simulink model "DigitalTwin"  (R2023b)
settings: Solver=ode23t  StartTime=0.0  StopTime=600  RelTol=1e-3  AbsTol=1e-3
model workspace: external: MATLAB File C:\Users\claud\OneDrive - TUM\COME -TUM\Software lab\Three_wheeled_base\simscape_1\Three_wheeled_base_DataFile1.m (data not in the file)
values from neighbouring files (symbols this model uses):
  brick_pick_global_xy = [brick_pick_global_xy, new_column]    [Three_wheeled_base_LOAD_DATA.m]
  brick_place_global_xy = [brick_place_global_xy, new_column]    [Three_wheeled_base_LOAD_DATA.m]
  platform_destination_mat = [ 1.0 0; 5 0; 0 0; 0 5 ... (first row only)    [Three_wheeled_base_LOAD_DATA.m]
undefined symbols (not defined in the file or in its folder): robotData, smiData, X, Y, Z
libraries: sm_lib x237, nesl_utility x78, fl_lib x12, batteryecm_lib x5, ee_lib x3, robotcorelib x1, robotalgslib x1
(part 7 of 7)

== system DigitalTwin/Arm/Kinova Gen3 Arm/right_inner_knuckle ==
  Inertia : sm_lib/Body Elements/Inertia  InertiaType=Custom  Mass=0.0110930853895903  MassUnits=kg  CenterOfMass=[0, 0, 0]  CenterOfMassUnits=m  MomentsOfInertia=[4.27134775939882e-06, 3.96548790524392e-06, 3.20325997634666e-06]  MomentsOfInertiaUnits=kg*m^2  ProductsOfInertia=[-8.45108024914164e-15, 1.77774229944246e-06, -8.53568456728898e-15]  ProductsOfInertiaUnits=kg*m^2  GraphicType=None  MarkerShape=Inertia  MarkerSize=20  GraphicVisPropType=SimpleVisualProperties  GraphicDiffuseColor=[0.5 0.5 0.5]  GraphicSpecularColor=[0.5 0.5 0.5 1.0]  GraphicAmbientColor=[0.15 0.15 0.15 1.0]  GraphicEmissiveColor=[0.0 0.0 0.0 1.0]  GraphicShininess=75  GraphicOpacity=1.0
  InertiaOriginTransform : sm_lib/Frames and Transforms/Rigid Transform  TranslationMethod=Cartesian  TranslationStandardOffset=0  TranslationStandardOffsetUnits=m  TranslationStandardAxis=+Z  TranslationCartesianOffset=[0.0168606186773776, 3.93808471820465e-10, 0.0226699950793434]  TranslationCartesianOffsetUnits=m  TranslationROffset=0  TranslationROffsetUnits=m  TranslationZOffset=0  TranslationZOffsetUnits=m  TranslationThetaOffset=0  TranslationThetaOffsetUnits=deg  RotationMethod=RotationSequence  RotationAngleUnits=deg  RotationStandardAxis=+Z  RotationAngle=0.0  RotationArbitraryAxis=[0 0 1]  FollAlignAxisA=+X  BaseAlignAxisA=+Y  FollAlignAxisB=+Y  BaseAlignAxisB=+Z  RotationSequenceAxes=BaseAxes  RotationSequence=XYZ  RotationSequenceAngles=[0, 0, 0]  RotationSequenceAnglesUnits=rad  RotationMatrix=[1 0 0; 0 1 0; 0 0 1]  Quaternion=[1 0 0 0]
  ReferenceFrame : sm_lib/Frames and Transforms/Reference Frame
  Visual : sm_lib/Body Elements/File Solid  ExtGeomFileName=Gripper85\inner_knuckle_fine.STL  UnitType=Custom  ExtGeomFileUnits=m  StepReaderType=HEX  ExportConvexHullGeometry=off  InertiaType=Custom  Mass=0  MassUnits=kg  CenterOfMass=[0, 0, 0]  CenterOfMassUnits=m  MomentsOfInertia=[0, 0, 0]  MomentsOfInertiaUnits=kg*m^2  ProductsOfInertia=[0, 0, 0]  ProductsOfInertiaUnits=kg*m^2  BasedOnType=DensityFromFile  Density=1000  DensityUnits=kg/m^3  DoExposeReferenceFrame=on  SerializedFrames=<Frames/>  GraphicType=FromGeometry  MarkerShape=Sphere  MarkerSize=10  GraphicVisPropType=SimpleVisualProperties  GraphicDiffuseColor=[0.1, 0.1, 0.1]  GraphicSpecularColor=[0.5 0.5 0.5 1.0]  GraphicAmbientColor=[0.15 0.15 0.15 1.0]  GraphicEmissiveColor=[0.0 0.0 0.0 1.0]  GraphicShininess=75  GraphicOpacity=1
  VisualOriginTransform : sm_lib/Frames and Transforms/Rigid Transform  TranslationMethod=Cartesian  TranslationStandardOffset=0  TranslationStandardOffsetUnits=m  TranslationStandardAxis=+Z  TranslationCartesianOffset=[0, 0, 0]  TranslationCartesianOffsetUnits=m  TranslationROffset=0  TranslationROffsetUnits=m  TranslationZOffset=0  TranslationZOffsetUnits=m  TranslationThetaOffset=0  TranslationThetaOffsetUnits=deg  RotationMethod=RotationSequence  RotationAngleUnits=deg  RotationStandardAxis=+Z  RotationAngle=0.0  RotationArbitraryAxis=[0 0 1]  FollAlignAxisA=+X  BaseAlignAxisA=+Y  FollAlignAxisB=+Y  BaseAlignAxisB=+Z  RotationSequenceAxes=BaseAxes  RotationSequence=XYZ  RotationSequenceAngles=[0, 0, 0]  RotationSequenceAnglesUnits=rad  RotationMatrix=[1 0 0; 0 1 0; 0 0 1]  Quaternion=[1 0 0 0]
  right_inner_finger_joint_AxisTransform : sm_lib/Frames and Transforms/Rigid Transform  TranslationMethod=Cartesian  TranslationStandardOffset=0  TranslationStandardOffsetUnits=m  TranslationStandardAxis=+Z  TranslationCartesianOffset=[0, 0, 0]  TranslationCartesianOffsetUnits=m  TranslationROffset=0  TranslationROffsetUnits=m  TranslationZOffset=0  TranslationZOffsetUnits=m  TranslationThetaOffset=0  TranslationThetaOffsetUnits=deg  RotationMethod=ArbitraryAxis  RotationAngleUnits=rad  RotationStandardAxis=+Z  RotationAngle=1.570796326794897  RotationArbitraryAxis=[-1, 0, 0]  FollAlignAxisA=+X  BaseAlignAxisA=+Y  FollAlignAxisB=+Y  BaseAlignAxisB=+Z  RotationSequenceAxes=FollowerAxes  RotationSequence=XYX  RotationSequenceAngles=[0 0 0]  RotationSequenceAnglesUnits=deg  RotationMatrix=[1 0 0; 0 1 0; 0 0 1]  Quaternion=[1 0 0 0]
  right_inner_finger_joint_OriginTransform : sm_lib/Frames and Transforms/Rigid Transform  TranslationMethod=Cartesian  TranslationStandardOffset=0  TranslationStandardOffsetUnits=m  TranslationStandardAxis=+Z  TranslationCartesianOffset=[0.0341060475457406, 0, 0.0458573878541688]  TranslationCartesianOffsetUnits=m  TranslationROffset=0  TranslationROffsetUnits=m  TranslationZOffset=0  TranslationZOffsetUnits=m  TranslationThetaOffset=0  TranslationThetaOffsetUnits=deg  RotationMethod=RotationSequence  RotationAngleUnits=deg  RotationStandardAxis=+Z  RotationAngle=0.0  RotationArbitraryAxis=[0 0 1]  FollAlignAxisA=+X  BaseAlignAxisA=+Y  FollAlignAxisB=+Y  BaseAlignAxisB=+Z  RotationSequenceAxes=BaseAxes  RotationSequence=XYZ  RotationSequenceAngles=[0, 0, 0]  RotationSequenceAnglesUnits=rad  RotationMatrix=[1 0 0; 0 1 0; 0 0 1]  Quaternion=[1 0 0 0]
  right_inner_knuckle_joint_AxisInvTransform : sm_lib/Frames and Transforms/Rigid Transform  TranslationMethod=Cartesian  TranslationStandardOffset=0  TranslationStandardOffsetUnits=m  TranslationStandardAxis=+Z  TranslationCartesianOffset=[0, 0, 0]  TranslationCartesianOffsetUnits=m  TranslationROffset=0  TranslationROffsetUnits=m  TranslationZOffset=0  TranslationZOffsetUnits=m  TranslationThetaOffset=0  TranslationThetaOffsetUnits=deg  RotationMethod=ArbitraryAxis  RotationAngleUnits=rad  RotationStandardAxis=+Z  RotationAngle=1.570796326794897  RotationArbitraryAxis=[-1, 0, 0]  FollAlignAxisA=+X  BaseAlignAxisA=+Y  FollAlignAxisB=+Y  BaseAlignAxisB=+Z  RotationSequenceAxes=FollowerAxes  RotationSequence=XYX  RotationSequenceAngles=[0 0 0]  RotationSequenceAnglesUnits=deg  RotationMatrix=[1 0 0; 0 1 0; 0 0 1]  Quaternion=[1 0 0 0]
  F : PMIOPort  Side=Left
  F1 : PMIOPort  Port=2  Side=Right
  connections:
  Inertia/RConn1 -- InertiaOriginTransform/RConn1
  ReferenceFrame/RConn1 -- InertiaOriginTransform/LConn1 -- right_inner_finger_joint_OriginTransform/LConn1 -- right_inner_knuckle_joint_AxisInvTransform/LConn1 -- VisualOriginTransform/LConn1
  Visual/RConn1 -- VisualOriginTransform/RConn1
  right_inner_finger_joint_AxisTransform/RConn1 -- F1/RConn1
  right_inner_finger_joint_AxisTransform/LConn1 -- right_inner_finger_joint_OriginTransform/RConn1
  right_inner_knuckle_joint_AxisInvTransform/RConn1 -- F/RConn1

== system DigitalTwin/Arm/Kinova Gen3 Arm/right_outer_finger ==
  Inertia : sm_lib/Body Elements/Inertia  InertiaType=Custom  Mass=0.0273093985570947  MassUnits=kg  CenterOfMass=[0, 0, 0]  CenterOfMassUnits=m  MomentsOfInertia=[8.52366028592721e-06, 6.91333280651081e-06, 2.24270431912283e-06]  MomentsOfInertiaUnits=kg*m^2  ProductsOfInertia=[7.37726682706417e-19, 3.18003675694284e-07, 3.41683380899422e-19]  ProductsOfInertiaUnits=kg*m^2  GraphicType=None  MarkerShape=Inertia  MarkerSize=20  GraphicVisPropType=SimpleVisualProperties  GraphicDiffuseColor=[0.5 0.5 0.5]  GraphicSpecularColor=[0.5 0.5 0.5 1.0]  GraphicAmbientColor=[0.15 0.15 0.15 1.0]  GraphicEmissiveColor=[0.0 0.0 0.0 1.0]  GraphicShininess=75  GraphicOpacity=1.0
  InertiaOriginTransform : sm_lib/Frames and Transforms/Rigid Transform  TranslationMethod=Cartesian  TranslationStandardOffset=0  TranslationStandardOffsetUnits=m  TranslationStandardAxis=+Z  TranslationCartesianOffset=[0.00108844269639009, -2.611488350845e-15, 0.0215530225245502]  TranslationCartesianOffsetUnits=m  TranslationROffset=0  TranslationROffsetUnits=m  TranslationZOffset=0  TranslationZOffsetUnits=m  TranslationThetaOffset=0  TranslationThetaOffsetUnits=deg  RotationMethod=RotationSequence  RotationAngleUnits=deg  RotationStandardAxis=+Z  RotationAngle=0.0  RotationArbitraryAxis=[0 0 1]  FollAlignAxisA=+X  BaseAlignAxisA=+Y  FollAlignAxisB=+Y  BaseAlignAxisB=+Z  RotationSequenceAxes=BaseAxes  RotationSequence=XYZ  RotationSequenceAngles=[0, 0, 0]  RotationSequenceAnglesUnits=rad  RotationMatrix=[1 0 0; 0 1 0; 0 0 1]  Quaternion=[1 0 0 0]
  ReferenceFrame : sm_lib/Frames and Transforms/Reference Frame
  Visual : sm_lib/Body Elements/File Solid  ExtGeomFileName=Gripper85\outer_finger_fine.STL  UnitType=Custom  ExtGeomFileUnits=m  StepReaderType=HEX  ExportConvexHullGeometry=off  InertiaType=Custom  Mass=0  MassUnits=kg  CenterOfMass=[0, 0, 0]  CenterOfMassUnits=m  MomentsOfInertia=[0, 0, 0]  MomentsOfInertiaUnits=kg*m^2  ProductsOfInertia=[0, 0, 0]  ProductsOfInertiaUnits=kg*m^2  BasedOnType=DensityFromFile  Density=1000  DensityUnits=kg/m^3  DoExposeReferenceFrame=on  SerializedFrames=<Frames/>  GraphicType=FromGeometry  MarkerShape=Sphere  MarkerSize=10  GraphicVisPropType=SimpleVisualProperties  GraphicDiffuseColor=[0.1, 0.1, 0.1]  GraphicSpecularColor=[0.5 0.5 0.5 1.0]  GraphicAmbientColor=[0.15 0.15 0.15 1.0]  GraphicEmissiveColor=[0.0 0.0 0.0 1.0]  GraphicShininess=75  GraphicOpacity=1
  VisualOriginTransform : sm_lib/Frames and Transforms/Rigid Transform  TranslationMethod=Cartesian  TranslationStandardOffset=0  TranslationStandardOffsetUnits=m  TranslationStandardAxis=+Z  TranslationCartesianOffset=[0, 0, 0]  TranslationCartesianOffsetUnits=m  TranslationROffset=0  TranslationROffsetUnits=m  TranslationZOffset=0  TranslationZOffsetUnits=m  TranslationThetaOffset=0  TranslationThetaOffsetUnits=deg  RotationMethod=RotationSequence  RotationAngleUnits=deg  RotationStandardAxis=+Z  RotationAngle=0.0  RotationArbitraryAxis=[0 0 1]  FollAlignAxisA=+X  BaseAlignAxisA=+Y  FollAlignAxisB=+Y  BaseAlignAxisB=+Z  RotationSequenceAxes=BaseAxes  RotationSequence=XYZ  RotationSequenceAngles=[0, 0, 0]  RotationSequenceAnglesUnits=rad  RotationMatrix=[1 0 0; 0 1 0; 0 0 1]  Quaternion=[1 0 0 0]
  F : PMIOPort  Side=Left
  connections:
  Inertia/RConn1 -- InertiaOriginTransform/RConn1
  ReferenceFrame/RConn1 -- InertiaOriginTransform/LConn1 -- VisualOriginTransform/LConn1 -- F/RConn1
  Visual/RConn1 -- VisualOriginTransform/RConn1

== system DigitalTwin/Arm/Kinova Gen3 Arm/right_outer_knuckle ==
  Inertia : sm_lib/Body Elements/Inertia  InertiaType=Custom  Mass=0.00684838849401352  MassUnits=kg  CenterOfMass=[0, 0, 0]  CenterOfMassUnits=m  MomentsOfInertia=[2.70004361573169e-07, 1.38892332558312e-06, 1.26286103637978e-06]  MomentsOfInertiaUnits=kg*m^2  ProductsOfInertia=[2.82357800318817e-15, 1.56396493788199e-07, 1.59579467624491e-15]  ProductsOfInertiaUnits=kg*m^2  GraphicType=None  MarkerShape=Inertia  MarkerSize=20  GraphicVisPropType=SimpleVisualProperties  GraphicDiffuseColor=[0.5 0.5 0.5]  GraphicSpecularColor=[0.5 0.5 0.5 1.0]  GraphicAmbientColor=[0.15 0.15 0.15 1.0]  GraphicEmissiveColor=[0.0 0.0 0.0 1.0]  GraphicShininess=75  GraphicOpacity=1.0
  InertiaOriginTransform : sm_lib/Frames and Transforms/Rigid Transform  TranslationMethod=Cartesian  TranslationStandardOffset=0  TranslationStandardOffsetUnits=m  TranslationStandardAxis=+Z  TranslationCartesianOffset=[0.0178097074051638, 3.60493211424024e-11, 0.00233123458346721]  TranslationCartesianOffsetUnits=m  TranslationROffset=0  TranslationROffsetUnits=m  TranslationZOffset=0  TranslationZOffsetUnits=m  TranslationThetaOffset=0  TranslationThetaOffsetUnits=deg  RotationMethod=RotationSequence  RotationAngleUnits=deg  RotationStandardAxis=+Z  RotationAngle=0.0  RotationArbitraryAxis=[0 0 1]  FollAlignAxisA=+X  BaseAlignAxisA=+Y  FollAlignAxisB=+Y  BaseAlignAxisB=+Z  RotationSequenceAxes=BaseAxes  RotationSequence=XYZ  RotationSequenceAngles=[0, 0, 0]  RotationSequenceAnglesUnits=rad  RotationMatrix=[1 0 0; 0 1 0; 0 0 1]  Quaternion=[1 0 0 0]
  ReferenceFrame : sm_lib/Frames and Transforms/Reference Frame
  Visual : sm_lib/Body Elements/File Solid  ExtGeomFileName=Gripper85\outer_knuckle_fine.STL  UnitType=Custom  ExtGeomFileUnits=m  StepReaderType=HEX  ExportConvexHullGeometry=off  InertiaType=Custom  Mass=0  MassUnits=kg  CenterOfMass=[0, 0, 0]  CenterOfMassUnits=m  MomentsOfInertia=[0, 0, 0]  MomentsOfInertiaUnits=kg*m^2  ProductsOfInertia=[0, 0, 0]  ProductsOfInertiaUnits=kg*m^2  BasedOnType=DensityFromFile  Density=1000  DensityUnits=kg/m^3  DoExposeReferenceFrame=on  SerializedFrames=<Frames/>  GraphicType=FromGeometry  MarkerShape=Sphere  MarkerSize=10  GraphicVisPropType=SimpleVisualProperties  GraphicDiffuseColor=[0.1, 0.1, 0.1]  GraphicSpecularColor=[0.5 0.5 0.5 1.0]  GraphicAmbientColor=[0.15 0.15 0.15 1.0]  GraphicEmissiveColor=[0.0 0.0 0.0 1.0]  GraphicShininess=75  GraphicOpacity=1
  VisualOriginTransform : sm_lib/Frames and Transforms/Rigid Transform  TranslationMethod=Cartesian  TranslationStandardOffset=0  TranslationStandardOffsetUnits=m  TranslationStandardAxis=+Z  TranslationCartesianOffset=[0, 0, 0]  TranslationCartesianOffsetUnits=m  TranslationROffset=0  TranslationROffsetUnits=m  TranslationZOffset=0  TranslationZOffsetUnits=m  TranslationThetaOffset=0  TranslationThetaOffsetUnits=deg  RotationMethod=RotationSequence  RotationAngleUnits=deg  RotationStandardAxis=+Z  RotationAngle=0.0  RotationArbitraryAxis=[0 0 1]  FollAlignAxisA=+X  BaseAlignAxisA=+Y  FollAlignAxisB=+Y  BaseAlignAxisB=+Z  RotationSequenceAxes=BaseAxes  RotationSequence=XYZ  RotationSequenceAngles=[0, 0, 0]  RotationSequenceAnglesUnits=rad  RotationMatrix=[1 0 0; 0 1 0; 0 0 1]  Quaternion=[1 0 0 0]
  right_outer_finger_joint_OriginTransform : sm_lib/Frames and Transforms/Rigid Transform  TranslationMethod=Cartesian  TranslationStandardOffset=0  TranslationStandardOffsetUnits=m  TranslationStandardAxis=+Z  TranslationCartesianOffset=[0.0317095909367246, 0, -0.0016013564954687]  TranslationCartesianOffsetUnits=m  TranslationROffset=0  TranslationROffsetUnits=m  TranslationZOffset=0  TranslationZOffsetUnits=m  TranslationThetaOffset=0  TranslationThetaOffsetUnits=deg  RotationMethod=RotationSequence  RotationAngleUnits=deg  RotationStandardAxis=+Z  RotationAngle=0.0  RotationArbitraryAxis=[0 0 1]  FollAlignAxisA=+X  BaseAlignAxisA=+Y  FollAlignAxisB=+Y  BaseAlignAxisB=+Z  RotationSequenceAxes=BaseAxes  RotationSequence=XYZ  RotationSequenceAngles=[0, 0, 0]  RotationSequenceAnglesUnits=rad  RotationMatrix=[1 0 0; 0 1 0; 0 0 1]  Quaternion=[1 0 0 0]
  right_outer_knuckle_joint_AxisInvTransform : sm_lib/Frames and Transforms/Rigid Transform  TranslationMethod=Cartesian  TranslationStandardOffset=0  TranslationStandardOffsetUnits=m  TranslationStandardAxis=+Z  TranslationCartesianOffset=[0, 0, 0]  TranslationCartesianOffsetUnits=m  TranslationROffset=0  TranslationROffsetUnits=m  TranslationZOffset=0  TranslationZOffsetUnits=m  TranslationThetaOffset=0  TranslationThetaOffsetUnits=deg  RotationMethod=ArbitraryAxis  RotationAngleUnits=rad  RotationStandardAxis=+Z  RotationAngle=1.570796326794897  RotationArbitraryAxis=[-1, 0, 0]  FollAlignAxisA=+X  BaseAlignAxisA=+Y  FollAlignAxisB=+Y  BaseAlignAxisB=+Z  RotationSequenceAxes=FollowerAxes  RotationSequence=XYX  RotationSequenceAngles=[0 0 0]  RotationSequenceAnglesUnits=deg  RotationMatrix=[1 0 0; 0 1 0; 0 0 1]  Quaternion=[1 0 0 0]
  F : PMIOPort  Side=Left
  F1 : PMIOPort  Port=2  Side=Right
  connections:
  Inertia/RConn1 -- InertiaOriginTransform/RConn1
  ReferenceFrame/RConn1 -- InertiaOriginTransform/LConn1 -- right_outer_finger_joint_OriginTransform/LConn1 -- right_outer_knuckle_joint_AxisInvTransform/LConn1 -- VisualOriginTransform/LConn1
  Visual/RConn1 -- VisualOriginTransform/RConn1
  right_outer_finger_joint_OriginTransform/RConn1 -- F1/RConn1
  right_outer_knuckle_joint_AxisInvTransform/RConn1 -- F/RConn1

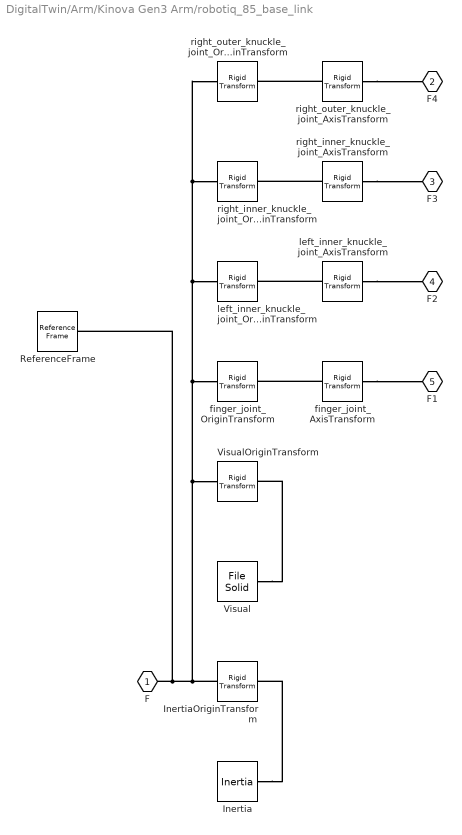
== system DigitalTwin/Arm/Kinova Gen3 Arm/robotiq_85_base_link ==
  Inertia : sm_lib/Body Elements/Inertia  InertiaType=Custom  Mass=0.30915  MassUnits=kg  CenterOfMass=[0, 0, 0]  CenterOfMassUnits=m  MomentsOfInertia=[0.00028972, 0.00030737, 0.00019914]  MomentsOfInertiaUnits=kg*m^2  ProductsOfInertia=[1.682e-12, -1.8543e-06, -5.7879e-10]  ProductsOfInertiaUnits=kg*m^2  GraphicType=None  MarkerShape=Inertia  MarkerSize=20  GraphicVisPropType=SimpleVisualProperties  GraphicDiffuseColor=[0.5 0.5 0.5]  GraphicSpecularColor=[0.5 0.5 0.5 1.0]  GraphicAmbientColor=[0.15 0.15 0.15 1.0]  GraphicEmissiveColor=[0.0 0.0 0.0 1.0]  GraphicShininess=75  GraphicOpacity=1.0
  InertiaOriginTransform : sm_lib/Frames and Transforms/Rigid Transform  TranslationMethod=Cartesian  TranslationStandardOffset=0  TranslationStandardOffsetUnits=m  TranslationStandardAxis=+Z  TranslationCartesianOffset=[0.00021987, -2.3546e-10, 0.030163]  TranslationCartesianOffsetUnits=m  TranslationROffset=0  TranslationROffsetUnits=m  TranslationZOffset=0  TranslationZOffsetUnits=m  TranslationThetaOffset=0  TranslationThetaOffsetUnits=deg  RotationMethod=RotationSequence  RotationAngleUnits=deg  RotationStandardAxis=+Z  RotationAngle=0.0  RotationArbitraryAxis=[0 0 1]  FollAlignAxisA=+X  BaseAlignAxisA=+Y  FollAlignAxisB=+Y  BaseAlignAxisB=+Z  RotationSequenceAxes=BaseAxes  RotationSequence=XYZ  RotationSequenceAngles=[0, 0, 0]  RotationSequenceAnglesUnits=rad  RotationMatrix=[1 0 0; 0 1 0; 0 0 1]  Quaternion=[1 0 0 0]
  ReferenceFrame : sm_lib/Frames and Transforms/Reference Frame
  Visual : sm_lib/Body Elements/File Solid  ExtGeomFileName=Gripper85\robotiq_85_base_link_fine.STL  UnitType=Custom  ExtGeomFileUnits=m  StepReaderType=HEX  ExportConvexHullGeometry=off  InertiaType=Custom  Mass=0  MassUnits=kg  CenterOfMass=[0, 0, 0]  CenterOfMassUnits=m  MomentsOfInertia=[0, 0, 0]  MomentsOfInertiaUnits=kg*m^2  ProductsOfInertia=[0, 0, 0]  ProductsOfInertiaUnits=kg*m^2  BasedOnType=DensityFromFile  Density=1000  DensityUnits=kg/m^3  DoExposeReferenceFrame=on  SerializedFrames=<Frames/>  GraphicType=FromGeometry  MarkerShape=Sphere  MarkerSize=10  GraphicVisPropType=SimpleVisualProperties  GraphicDiffuseColor=[0.1, 0.1, 0.1]  GraphicSpecularColor=[0.5 0.5 0.5 1.0]  GraphicAmbientColor=[0.15 0.15 0.15 1.0]  GraphicEmissiveColor=[0.0 0.0 0.0 1.0]  GraphicShininess=75  GraphicOpacity=1
  VisualOriginTransform : sm_lib/Frames and Transforms/Rigid Transform  TranslationMethod=Cartesian  TranslationStandardOffset=0  TranslationStandardOffsetUnits=m  TranslationStandardAxis=+Z  TranslationCartesianOffset=[0, 0, 0]  TranslationCartesianOffsetUnits=m  TranslationROffset=0  TranslationROffsetUnits=m  TranslationZOffset=0  TranslationZOffsetUnits=m  TranslationThetaOffset=0  TranslationThetaOffsetUnits=deg  RotationMethod=RotationSequence  RotationAngleUnits=deg  RotationStandardAxis=+Z  RotationAngle=0.0  RotationArbitraryAxis=[0 0 1]  FollAlignAxisA=+X  BaseAlignAxisA=+Y  FollAlignAxisB=+Y  BaseAlignAxisB=+Z  RotationSequenceAxes=BaseAxes  RotationSequence=XYZ  RotationSequenceAngles=[0, 0, 0]  RotationSequenceAnglesUnits=rad  RotationMatrix=[1 0 0; 0 1 0; 0 0 1]  Quaternion=[1 0 0 0]
  finger_joint_AxisTransform : sm_lib/Frames and Transforms/Rigid Transform  TranslationMethod=Cartesian  TranslationStandardOffset=0  TranslationStandardOffsetUnits=m  TranslationStandardAxis=+Z  TranslationCartesianOffset=[0, 0, 0]  TranslationCartesianOffsetUnits=m  TranslationROffset=0  TranslationROffsetUnits=m  TranslationZOffset=0  TranslationZOffsetUnits=m  TranslationThetaOffset=0  TranslationThetaOffsetUnits=deg  RotationMethod=ArbitraryAxis  RotationAngleUnits=rad  RotationStandardAxis=+Z  RotationAngle=1.570796326794897  RotationArbitraryAxis=[1, 0, 0]  FollAlignAxisA=+X  BaseAlignAxisA=+Y  FollAlignAxisB=+Y  BaseAlignAxisB=+Z  RotationSequenceAxes=FollowerAxes  RotationSequence=XYX  RotationSequenceAngles=[0 0 0]  RotationSequenceAnglesUnits=deg  RotationMatrix=[1 0 0; 0 1 0; 0 0 1]  Quaternion=[1 0 0 0]
  finger_joint_OriginTransform : sm_lib/Frames and Transforms/Rigid Transform  TranslationMethod=Cartesian  TranslationStandardOffset=0  TranslationStandardOffsetUnits=m  TranslationStandardAxis=+Z  TranslationCartesianOffset=[0.0306011444260539, 0, 0.06279201626953949]  TranslationCartesianOffsetUnits=m  TranslationROffset=0  TranslationROffsetUnits=m  TranslationZOffset=0  TranslationZOffsetUnits=m  TranslationThetaOffset=0  TranslationThetaOffsetUnits=deg  RotationMethod=RotationSequence  RotationAngleUnits=deg  RotationStandardAxis=+Z  RotationAngle=0.0  RotationArbitraryAxis=[0 0 1]  FollAlignAxisA=+X  BaseAlignAxisA=+Y  FollAlignAxisB=+Y  BaseAlignAxisB=+Z  RotationSequenceAxes=BaseAxes  RotationSequence=XYZ  RotationSequenceAngles=[0, 0, 0]  RotationSequenceAnglesUnits=rad  RotationMatrix=[1 0 0; 0 1 0; 0 0 1]  Quaternion=[1 0 0 0]
  left_inner_knuckle_joint_AxisTransform : sm_lib/Frames and Transforms/Rigid Transform  TranslationMethod=Cartesian  TranslationStandardOffset=0  TranslationStandardOffsetUnits=m  TranslationStandardAxis=+Z  TranslationCartesianOffset=[0, 0, 0]  TranslationCartesianOffsetUnits=m  TranslationROffset=0  TranslationROffsetUnits=m  TranslationZOffset=0  TranslationZOffsetUnits=m  TranslationThetaOffset=0  TranslationThetaOffsetUnits=deg  RotationMethod=ArbitraryAxis  RotationAngleUnits=rad  RotationStandardAxis=+Z  RotationAngle=1.570796326794897  RotationArbitraryAxis=[1, 0, 0]  FollAlignAxisA=+X  BaseAlignAxisA=+Y  FollAlignAxisB=+Y  BaseAlignAxisB=+Z  RotationSequenceAxes=FollowerAxes  RotationSequence=XYX  RotationSequenceAngles=[0 0 0]  RotationSequenceAnglesUnits=deg  RotationMatrix=[1 0 0; 0 1 0; 0 0 1]  Quaternion=[1 0 0 0]
  left_inner_knuckle_joint_OriginTransform : sm_lib/Frames and Transforms/Rigid Transform  TranslationMethod=Cartesian  TranslationStandardOffset=0  TranslationStandardOffsetUnits=m  TranslationStandardAxis=+Z  TranslationCartesianOffset=[0.0127000000001501, 0, 0.0693074999999639]  TranslationCartesianOffsetUnits=m  TranslationROffset=0  TranslationROffsetUnits=m  TranslationZOffset=0  TranslationZOffsetUnits=m  TranslationThetaOffset=0  TranslationThetaOffsetUnits=deg  RotationMethod=RotationSequence  RotationAngleUnits=deg  RotationStandardAxis=+Z  RotationAngle=0.0  RotationArbitraryAxis=[0 0 1]  FollAlignAxisA=+X  BaseAlignAxisA=+Y  FollAlignAxisB=+Y  BaseAlignAxisB=+Z  RotationSequenceAxes=BaseAxes  RotationSequence=XYZ  RotationSequenceAngles=[0, 0, 0]  RotationSequenceAnglesUnits=rad  RotationMatrix=[1 0 0; 0 1 0; 0 0 1]  Quaternion=[1 0 0 0]
  right_inner_knuckle_joint_AxisTransform : sm_lib/Frames and Transforms/Rigid Transform  TranslationMethod=Cartesian  TranslationStandardOffset=0  TranslationStandardOffsetUnits=m  TranslationStandardAxis=+Z  TranslationCartesianOffset=[0, 0, 0]  TranslationCartesianOffsetUnits=m  TranslationROffset=0  TranslationROffsetUnits=m  TranslationZOffset=0  TranslationZOffsetUnits=m  TranslationThetaOffset=0  TranslationThetaOffsetUnits=deg  RotationMethod=ArbitraryAxis  RotationAngleUnits=rad  RotationStandardAxis=+Z  RotationAngle=1.570796326794897  RotationArbitraryAxis=[-1, 0, 0]  FollAlignAxisA=+X  BaseAlignAxisA=+Y  FollAlignAxisB=+Y  BaseAlignAxisB=+Z  RotationSequenceAxes=FollowerAxes  RotationSequence=XYX  RotationSequenceAngles=[0 0 0]  RotationSequenceAnglesUnits=deg  RotationMatrix=[1 0 0; 0 1 0; 0 0 1]  Quaternion=[1 0 0 0]
  right_inner_knuckle_joint_OriginTransform : sm_lib/Frames and Transforms/Rigid Transform  TranslationMethod=Cartesian  TranslationStandardOffset=0  TranslationStandardOffsetUnits=m  TranslationStandardAxis=+Z  TranslationCartesianOffset=[-0.0126999999998499, 0, 0.0693075000000361]  TranslationCartesianOffsetUnits=m  TranslationROffset=0  TranslationROffsetUnits=m  TranslationZOffset=0  TranslationZOffsetUnits=m  TranslationThetaOffset=0  TranslationThetaOffsetUnits=deg  RotationMethod=RotationSequence  RotationAngleUnits=deg  RotationStandardAxis=+Z  RotationAngle=0.0  RotationArbitraryAxis=[0 0 1]  FollAlignAxisA=+X  BaseAlignAxisA=+Y  FollAlignAxisB=+Y  BaseAlignAxisB=+Z  RotationSequenceAxes=BaseAxes  RotationSequence=XYZ  RotationSequenceAngles=[0, 0, 3.14159265358979]  RotationSequenceAnglesUnits=rad  RotationMatrix=[1 0 0; 0 1 0; 0 0 1]  Quaternion=[1 0 0 0]
  right_outer_knuckle_joint_AxisTransform : sm_lib/Frames and Transforms/Rigid Transform  TranslationMethod=Cartesian  TranslationStandardOffset=0  TranslationStandardOffsetUnits=m  TranslationStandardAxis=+Z  TranslationCartesianOffset=[0, 0, 0]  TranslationCartesianOffsetUnits=m  TranslationROffset=0  TranslationROffsetUnits=m  TranslationZOffset=0  TranslationZOffsetUnits=m  TranslationThetaOffset=0  TranslationThetaOffsetUnits=deg  RotationMethod=ArbitraryAxis  RotationAngleUnits=rad  RotationStandardAxis=+Z  RotationAngle=1.570796326794897  RotationArbitraryAxis=[-1, 0, 0]  FollAlignAxisA=+X  BaseAlignAxisA=+Y  FollAlignAxisB=+Y  BaseAlignAxisB=+Z  RotationSequenceAxes=FollowerAxes  RotationSequence=XYX  RotationSequenceAngles=[0 0 0]  RotationSequenceAnglesUnits=deg  RotationMatrix=[1 0 0; 0 1 0; 0 0 1]  Quaternion=[1 0 0 0]
  right_outer_knuckle_joint_OriginTransform : sm_lib/Frames and Transforms/Rigid Transform  TranslationMethod=Cartesian  TranslationStandardOffset=0  TranslationStandardOffsetUnits=m  TranslationStandardAxis=+Z  TranslationCartesianOffset=[-0.0306011444258893, 0, 0.06279201626953949]  TranslationCartesianOffsetUnits=m  TranslationROffset=0  TranslationROffsetUnits=m  TranslationZOffset=0  TranslationZOffsetUnits=m  TranslationThetaOffset=0  TranslationThetaOffsetUnits=deg  RotationMethod=RotationSequence  RotationAngleUnits=deg  RotationStandardAxis=+Z  RotationAngle=0.0  RotationArbitraryAxis=[0 0 1]  FollAlignAxisA=+X  BaseAlignAxisA=+Y  FollAlignAxisB=+Y  BaseAlignAxisB=+Z  RotationSequenceAxes=BaseAxes  RotationSequence=XYZ  RotationSequenceAngles=[0, 0, 3.14159265358979]  RotationSequenceAnglesUnits=rad  RotationMatrix=[1 0 0; 0 1 0; 0 0 1]  Quaternion=[1 0 0 0]
  F : PMIOPort  Side=Left
  F4 : PMIOPort  Port=2  Side=Right
  F3 : PMIOPort  Port=3  Side=Right
  F2 : PMIOPort  Port=4  Side=Right
  F1 : PMIOPort  Port=5  Side=Right
  connections:
  Inertia/RConn1 -- InertiaOriginTransform/RConn1
  ReferenceFrame/RConn1 -- InertiaOriginTransform/LConn1 -- right_inner_knuckle_joint_OriginTransform/LConn1 -- right_outer_knuckle_joint_OriginTransform/LConn1 -- left_inner_knuckle_joint_OriginTransform/LConn1 -- finger_joint_OriginTransform/LConn1 -- VisualOriginTransform/LConn1 -- F/RConn1
  Visual/RConn1 -- VisualOriginTransform/RConn1
  finger_joint_AxisTransform/RConn1 -- F1/RConn1
  finger_joint_AxisTransform/LConn1 -- finger_joint_OriginTransform/RConn1
  left_inner_knuckle_joint_AxisTransform/RConn1 -- F2/RConn1
  left_inner_knuckle_joint_AxisTransform/LConn1 -- left_inner_knuckle_joint_OriginTransform/RConn1
  right_inner_knuckle_joint_AxisTransform/RConn1 -- F3/RConn1
  right_inner_knuckle_joint_AxisTransform/LConn1 -- right_inner_knuckle_joint_OriginTransform/RConn1
  right_outer_knuckle_joint_AxisTransform/RConn1 -- F4/RConn1
  right_outer_knuckle_joint_AxisTransform/LConn1 -- right_outer_knuckle_joint_OriginTransform/RConn1

== matlab function DigitalTwin/Task Scheduler ==
  data: platform_xy input; platform_orientation input; platformWaypoints output; platform_mode_out output; reset_time_out_arm output; arm_waypoints output; endtime_out output; arm_mode_out output; it_brick_out output; stop_simulation output; current_time input; brick_pick_relative input; brick_place_global_xy input; platform_destination_mat input
function [platformWaypoints,platform_mode_out, reset_time_out_arm,arm_waypoints, endtime_out,arm_mode_out, it_brick_out,stop_simulation] ...
    = task_scheduler(platform_xy,platform_orientation, current_time, brick_pick_relative, brick_place_global_xy, platform_destination_mat)

%-------------- Inputs ------------------------------------------------------
% platform_xy: Platform position with respect to origin of mobile base plane
% platform_orientation: Angle which descirbes the orientation of the platform 
% current_time: Current time
% brick_pick_relative: Relative position of brick with respect to robotic arm
% brick_place_global_xy: Positions to place bricks with respect to origin of mobile base plane
% platform_destination_mat: Matrix containing the waypoints to generate path for the mobile base place

%-------------- Outputs ------------------------------------------------------
%platformWaypoints: Waypoints for the mobile base
%platform_mode_out: Mode of the platform
%reset_time_out_arm: Variable used to reset the time in trapezoidal velocity profile path function
%arm_waypoints: Waypoints between two consecutive poses of the robotic arm
%endtime_out: Time in order to complete a move between two consecutive poses
%arm_mode_out: arm mode 
%it_brick_out: Brick iterator used to stop the simulation weld join activation
%stop_simulation: Stop simulation when placed the third brick 

%-------------- Platform initialization  -----------------------------------------------------------------------
pickandplace_map = [2 4 6 8 10 12]; 
% Instances 2,6,10 are pick instances
% Instances 4,8,12 are pick instances
persistent previous_platform_position previous_platform_waypoints platform_destination
persistent  it_destination platform_move_begin platform_mode

if isempty(it_destination) 
    it_destination = 1; %Destination iterator
    platform_destination = platform_destination_mat(1,:); %First destination
end

if isempty(platform_move_begin) 
    platform_move_begin = 1;
    platform_mode = 0;
end
if isempty(previous_platform_waypoints) 
    previous_platform_waypoints = zeros(2,2);
end
if isempty(previous_platform_position)
    previous_platform_position = zeros(1,2);
end

platformWaypoints=previous_platform_waypoints;

%-------------- End of platform initialization -----------------------------------------------------------------

%-------------- Arm initialization  -------------------------------------------------------------------------
brick_above = [0 0 0.4]; % Approach the brick before picking 
brick_grip_pos = [0 0 0.175]; % Move vertically downward
persistent it_brick  arm_mode  reset_time_arm arm_move_finished previous_Arm_Waypoints total_Arm_Waypoints end_time 
if isempty(it_brick)
    it_brick = 1 ; %Brick iterator
end
if isempty(previous_Arm_Waypoints) 
    previous_Arm_Waypoints = zeros(8,2);
    total_Arm_Waypoints = zeros(8,9);
end
if isempty(arm_mode) 
    arm_mode = 0;
    end_time = 3;
end
if isempty(reset_time_arm) 
    reset_time_arm = 0;
end
if isempty(arm_move_finished)
    arm_move_finished = 1 ;
end
coder.extrinsic("sm_kinovaGen3_arm_ik");
eeIgs = zeros(1,7);
%-------------- End of arm initialization -------------------------------------------------------------------

%-------------- Platform TS  -----------------------------------------------------------------------
distanceToRun = norm(platform_destination - platform_xy'); % Distance to reach the goal

% Platform_move_begin = 1 is a command to start the mobile platform
% Arm mode 0,6,11 are modes where the arm is idle and the mobile platform can move
% When the robotic arm is at mode 5 or 10, arm mode is changed to 6 or 11 but its current task is still going on
% current_time - reset_time_arm > end_time + 0.1 -> makes sure that the arm has finished its current task
% it_destination <= size(platform_destination_mat,1) -> Iterator has reach the last destination
if platform_move_begin == 1 && (arm_mode == 0 || (arm_mode == 6 && current_time - reset_time_arm > end_time + 0.1 ) ...
    || (arm_mode == 11 && current_time - reset_time_arm > end_time + 0.1 ) ) && it_destination <= size(platform_destination_mat,1)
    
    disp("Entered platform scheduler")
    platform_move_begin = 0;
    platform_mode = 1;
    
    if  ismember(pickandplace_map(it_destination), pickandplace_map(1:2:end)) % Odd instances of pickandplace_map are for picking
        platformWaypoints(1,:) = platform_destination_mat(pickandplace_map(it_destination)-1,:); %Get new platformWaypoints
        platformWaypoints(2,:) = platform_destination_mat(pickandplace_map(it_destination)  ,:); %Get new platformWaypoints
        platform_destination = platformWaypoints(2,:); %Platform destination is the last platformWaypoint

        
        distanceToRun = norm(platform_destination - platform_xy');
        disp("Mobile base started towards brick picking location at time: ")
        disp(current_time)
        disp("Platform waypoints are: ")
        disp(platformWaypoints)
        disp("Platform destination is")
        disp(platform_destination)

    elseif ismember (pickandplace_map(it_destination), pickandplace_map(2:2:end) ) % Even instances of pickandplace_map are for placing
        platformWaypoints(1,:) = platform_destination_mat(pickandplace_map(it_destination)-1,:); %Get new platformWaypoints
        platformWaypoints(2,:) = platform_destination_mat(pickandplace_map(it_destination)  ,:); %Get new platformWaypoints
        platform_destination = platformWaypoints(2,:); %Platform destination is the last platformWaypoint

        disp("Platform destination is")
        disp(platform_destination)
        distanceToRun = norm(platform_destination - platform_xy');
        disp("Mobile base started after picked brick at time: ")
        disp(current_time)
        disp("Platform waypoints are: ")
        disp(platformWaypoints)
        disp("Platform destination is")
        disp(platform_destination)

    end  

    if size(platform_destination_mat,1) >= it_destination 
            it_destination = it_destination + 1; 
    end

    previous_platform_waypoints = platformWaypoints;
    previous_platform_position = platform_destination;

end


if (platform_mode == 1) && distanceToRun<=0.01 % Platform is near the destination
    disp("Mobile base movement finished at time")
    disp(current_time)
    disp("Mobile base origin is at ")
    disp(platform_xy)
    platform_mode = 0 ;
    if arm_mode == 0 || arm_mode == 11 %Gripper is empty and must start picking a brick
        arm_mode = 1 ;
        previous_Arm_Waypoints = zeros(8,2);
        reset_time_arm =  current_time;
        end_time = 3;
    elseif arm_mode == 6 %Gripper has a brick and must start placing it 
        arm_mode = 7 ;
    end        

end
%-------------- End of platform TS  -----------------------------------------------------------------------

%-------------- Arm TS  -----------------------------------------------------------------------
if it_brick <=3 %Task scheduler designed to pick and palce 3 bricks
relative_pick_pos = zeros(1,3);
relative_place_pos = zeros(1,3);
x_unrotated =  (brick_pick_relative(it_brick,1) );
y_unrotated =  (brick_pick_relative(it_brick,2) );
% Calculate correct position and orientation of the arm with respect to the brick for pick or place positions
relative_pick_pos(1) =  x_unrotated * cos(-platform_orientation) - y_unrotated * sin(-platform_orientation) ;
relative_pick_pos(2) =  x_unrotated * sin(-platform_orientation) + y_unrotated * cos(-platform_orientation) ;
relative_pick_pos(3) = -0.033;
relative_place_pos(2) =  (brick_place_global_xy(it_brick,1) - platform_xy(1));
relative_place_pos(1) =  (brick_place_global_xy(it_brick,2) - platform_xy(2));
relative_place_pos(3) = brick_place_global_xy(it_brick,3);
else %After pick and place of the 3rd brick stay idle until simulation closes
    arm_mode = 12;  
    relative_place_pos = zeros(1,3);
    relative_pick_pos = zeros(1,3);
end

if arm_mode == 1  && current_time - reset_time_arm > end_time + 0.1
    arm_mode = 2 ;
    disp("Arm started approaching to pick at time")
    disp(current_time)
    disp("Brick is located wrt arm origin is")
    disp(relative_pick_pos)
    %TR_frame contains the (x,y,z) coordinates where we want to place the end effector thats
    TR_frame = [
    [relative_pick_pos+brick_above,[180 0 platform_orientation*(180/pi)]];... % Approach from above
    [relative_pick_pos+brick_grip_pos,[180 0 platform_orientation*(180/pi)]];... %Ready to pick
    [relative_pick_pos+brick_grip_pos,[180 0 platform_orientation*(180/pi)]];... %Picked brick
    [relative_pick_pos+brick_above,[180 0 platform_orientation*(180/pi)]] ];... % Go above again
    [solution,solvedFlag] =  sm_kinovaGen3_arm_ik(TR_frame,eeIgs);
    %total_Arm_Waypoints contain the different poses which are calculated from inverse kinematics
    total_Arm_Waypoints(1:7,:) = [zeros(7,1) solution zeros(7,4)];
    total_Arm_Waypoints(1:7,2:size(TR_frame,1)+1) = total_Arm_Waypoints(1:7,2:size(TR_frame,1)+1)./180*pi;
    total_Arm_Waypoints(8,1:3)=0.0; %Grip is open
    total_Arm_Waypoints(8,4:5)= 0.4;%Grip is engaged

    previous_Arm_Waypoints = total_Arm_Waypoints(:,1:2);
    reset_time_arm = current_time ;
    end_time = 5;
elseif arm_mode == 2 && current_time - reset_time_arm > end_time + 0.1
    disp("Arm started going down to pick at time")
    disp(current_time)
    arm_mode = 3;
  
    previous_Arm_Waypoints(:,1) = previous_Arm_Waypoints(:,2);
    previous_Arm_Waypoints(:,2) = total_Arm_Waypoints(:,3);
    reset_time_arm = current_time ;
    end_time = 2.0;
elseif arm_mode == 3 && current_time - reset_time_arm > end_time + 0.1
    disp("Arm started closing grips to pick at time")
    disp(current_time)
    arm_mode = 4;
    previous_Arm_Waypoints(:,1) = previous_Arm_Waypoints(:,2);
    previous_Arm_Waypoints(:,2) = total_Arm_Waypoints(:,4);
    reset_time_arm = current_time ;
    end_time = 1.0;
elseif arm_mode == 4 && current_time - reset_time_arm > end_time + 0.1
    arm_mode = 5;
    disp("Arm picked and the gripper started moving a bit higher")
    disp(current_time)
    previous_Arm_Waypoints(:,1) = previous_Arm_Waypoints(:,2);
    previous_Arm_Waypoints(:,2) = total_Arm_Waypoints(:,5);

    reset_time_arm = current_time ;
    end_time = 2.0;
elseif arm_mode == 5 && current_time - reset_time_arm > end_time + 0.1
    disp("Arm start moving to the highest position")
    disp(current_time)
    arm_mode = 6;
    platform_move_begin = 1;
    previous_Arm_Waypoints(:,1) = previous_Arm_Waypoints(:,2);
    previous_Arm_Waypoints(1:7,2) = zeros(7,1);
    reset_time_arm = current_time ;
    end_time = 5.0;
elseif arm_mode == 7 && current_time  - reset_time_arm > end_time + 0.1
    arm_mode = 8;
    disp("Arm started approaching to place the brick at time")
    disp(current_time)
    disp("Place that brick will be placed wrt arm origin is ")
    disp(relative_place_pos)     
    
    TR_frame = [
    [relative_place_pos+brick_grip_pos, [180 0 platform_orientation*(180/pi)-90]];...
    [relative_place_pos+brick_grip_pos, [180 0 platform_orientation*(180/pi)-90]];...
    [relative_place_pos+brick_above,    [180 0 platform_orientation*(180/pi)-90]]];
    [solution] =  sm_kinovaGen3_arm_ik(TR_frame,eeIgs);
    total_Arm_Waypoints(1:7,6:8) = solution./180*pi; 
    total_Arm_Waypoints(8,6)= 0.2;
    total_Arm_Waypoints(8,7:8) = -0.3;
    previous_Arm_Waypoints(:,1) = previous_Arm_Waypoints(:,2);
    previous_Arm_Waypoints(:,2) = total_Arm_Waypoints(:,6);
    reset_time_arm = current_time ;
    end_time = 5.0;
 elseif arm_mode == 8 && current_time - reset_time_arm > end_time + 0.1
    disp("Arm opened grips")
    disp(current_time)
    arm_mode = 9;
    previous_Arm_Waypoints(:,1) = previous_Arm_Waypoints(:,2);
    previous_Arm_Waypoints(:,2) = total_Arm_Waypoints(:,7);
    reset_time_arm = current_time ;
    end_time = 1.0;
  elseif arm_mode == 9 && current_time - reset_time_arm > end_time + 0.1
    disp("Arm went upper after it left the brick")
    disp(current_time)
    arm_mode = 10;
    previous_Arm_Waypoints(:,1) = previous_Arm_Waypoints(:,2);
    previous_Arm_Waypoints(:,2) = total_Arm_Waypoints(:,8);
    reset_time_arm = current_time ;
    end_time = 2.0;
  elseif arm_mode == 10 && current_time - reset_time_arm > end_time + 0.1
    disp("Arm went initial position")
    disp(current_time)
    platform_move_begin = 1;
    arm_mode = 11;
    previous_Arm_Waypoints(:,1) = previous_Arm_Waypoints(:,2);
    previous_Arm_Waypoints(:,2) = total_Arm_Waypoints(:,9);
    reset_time_arm = current_time ;
    end_time = 5;
    it_brick = it_brick + 1;
end

if arm_mode >= 5 && arm_mode <= 8 %Activate weld joint between for the brick
    WS_switch = 0;
else
    WS_switch = -1;
end

arm_mode_out = arm_mode;
it_brick_out = it_brick;

reset_time_out_arm = reset_time_arm ;
arm_waypoints = previous_Arm_Waypoints;
endtime_out = end_time;
platform_mode_out = platform_mode;
stop_simulation = 0;

if arm_mode ==12 && current_time - reset_time_arm > end_time + 0.1
    stop_simulation = 1;
end
%-------------- End of TS  --------------------------------------------------------------------

end

== matlab function DigitalTwin/Subsystem/Control/MATLAB Function ==
  data: goal_wL output; goal_wR output; xy input; target_position input; platform_mode_out input; velocity input; ang_vel input; distanceToRun output; velocity_out output
function [goal_wL, goal_wR, distanceToRun,velocity_out] = wheelVelocity(xy,target_position,platform_mode_out, velocity, ang_vel)
    wheelRadius=0.08;
    trackWidth=0.6124;
    stop = 0;
    % Slow the robot down when it's near the threshold with triangular
    % velocity profile
    distanceToRun = norm(target_position(end, :) - xy');
    distance_to_stop = 5*0.25/2;
    if distanceToRun <= distance_to_stop 
        velocity = sqrt(velocity^2 + (0-velocity)/(5)*2*(distance_to_stop -  distanceToRun)) ;
    end
    %Convert velocity to angular velocity in the wheels
    if platform_mode_out == 0  %%(distanceToRun<slowThreshold)
        velocity = 0;
        stop = 1;
        
    end

    velocity_out = velocity;
    goal_wL = +((velocity - trackWidth/2*ang_vel)/wheelRadius)*25/23*(1-stop);
    goal_wR = -((velocity + trackWidth/2*ang_vel)/wheelRadius)*25/23*(1-stop);
end

== matlab function DigitalTwin/Subsystem/Control/MATLAB Function1 ==
  settings: updateMethod=DISCRETE
  data: goal_wL output; goal_wR output; xy input; target_position input; velocity input; ang_vel input; distanceToRun output; current_time input; velocity_out output
function [goal_wL, goal_wR, distanceToRun,velocity_out] = wheelVelocity(xy,target_position,velocity, ang_vel, current_time)
    wheelRadius=0.06;
    slowThreshold= 2;  %Distance to target where velocity should be reduced
    stopThreshold=0.1; %Target reached
    trackWidth=0.0925;
    stop = 1;
    % Slow the robot down when it's near the threshold
    distanceToRun = norm(target_position(end, :) - xy');
    persistent trig_time slowmove_beg
    if isempty(trig_time)
        trig_time = 0;
        slowmove_beg = 1;
    end
    %Wheel speed computation
        %Slow base when it is close to the target
    if (distanceToRun<slowThreshold)
        if slowmove_beg == 1
            slowmove_beg = 0;
            trig_time = current_time;
        end
        velocity= 0.1 - (0.1 / 4)*(current_time - trig_time);
            %Stop base when it is in the target area
        if (distanceToRun<=stopThreshold)
            slowmove_beg = 1;
            stop = 0;
        end
    end
        %Convert velocity to angular velocity in the wheels
    velocity_out = velocity;
    goal_wL = +((velocity - trackWidth/2*ang_vel)/wheelRadius)*stop;
    goal_wR = -((velocity + trackWidth/2*ang_vel)/wheelRadius)*stop;
end

== matlab function DigitalTwin/Arm/Kinova Gen3 Arm/MATLAB Function ==
  data: arm_mode input; mode1 output; brick_iterator input; mode2 output; mode3 output
function [mode1,mode2,mode3]= fcn(arm_mode,brick_iterator)
mode1 = -1;
mode2 = -1;
mode3 = -1;
if arm_mode >= 5 && arm_mode <= 9 
    if brick_iterator == 1
        mode1 = 0;
    elseif brick_iterator == 2
        mode2 = 0;
    elseif brick_iterator == 3
        mode3 = 0;
    end
    
end
end
